simulink model "EjemploWebcam"  (Simulink 8.4)
settings: Solver=ode3  StartTime=0.0  StopTime=inf  FixedStep=0.001  RelTol=1e-3
libraries: rtwinlib x1
settings Model: Creator=Usuario  LastModifiedBy=Doc Avalos
settings OptimizationCC: SimCompilerOptimization=On

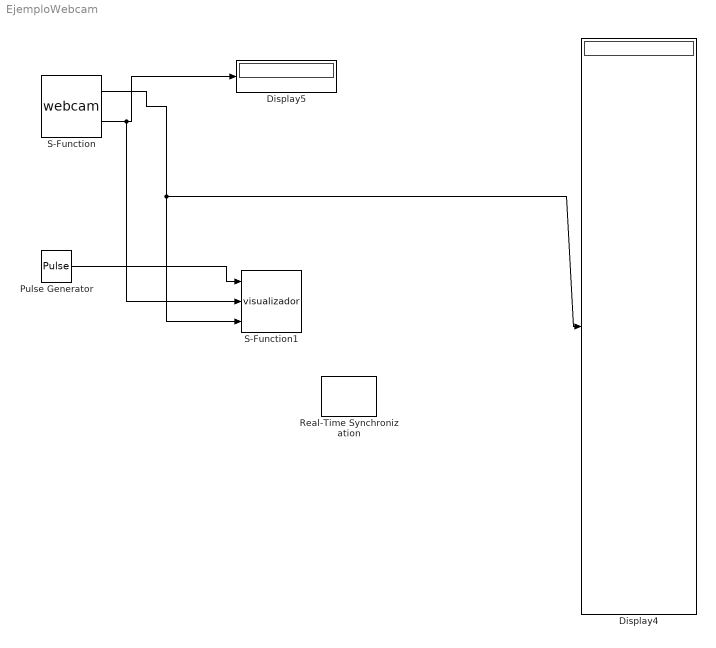
== system EjemploWebcam ==
  Display4 : Display
  Display5 : Display
  Pulse Generator : DiscretePulseGenerator  PulseType=Time based  Period=0.01  PulseWidth=50
  Real-Time Synchronization : rtwinlib/Real-Time Synchronization  SampleTime=0.1  MaxMissedTicks=inf  ShowMissedTicks=off  YieldWhenWaiting=off
  S-Function : S-Function  FunctionName=webcam  Parameters=1  EnableBusSupport=off
  S-Function1 : S-Function  FunctionName=visualizador  Parameters=1  EnableBusSupport=off
  wires:
  S-Function/1 -> S-Function1/3, Display4/1
  S-Function/2 -> Display5/1, S-Function1/2
  Pulse Generator/1 -> S-Function1/1
